simulink model "RobotArm_illinois"  (R2020a)
settings: Solver=VariableStepAuto  StartTime=0.0  StopTime=10.0  RelTol=1e-3
settings Model: Creator=nikhil  LastModifiedBy=nikhil

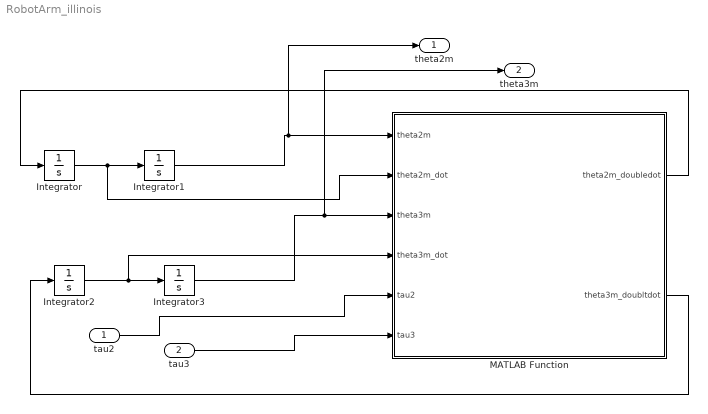
== system RobotArm_illinois ==
  tau2 : Inport
  tau3 : Inport  Port=2
  Integrator{,1..3} (4 alike) : Integrator
  MATLAB Function : MATLAB Function  TreatAsAtomicUnit=on
  theta2m : Outport
  theta3m : Outport  Port=2
  wires:
  Integrator/1 -> MATLAB Function/2(theta2m_dot), Integrator1/1
  Integrator2/1 -> MATLAB Function/4(theta3m_dot), Integrator3/1
  Integrator1/1 -> theta2m/1, MATLAB Function/1(theta2m)
  Integrator3/1 -> theta3m/1, MATLAB Function/3(theta3m)
  tau2/1 -> MATLAB Function/5(tau2)
  tau3/1 -> MATLAB Function/6(tau3)
  MATLAB Function/2(theta3m_doubltdot) -> Integrator2/1
  MATLAB Function/1(theta2m_doubledot) -> Integrator/1

== matlab function RobotArm_illinois/MATLAB Function ==
  data: theta2m input; theta2m_doubledot output; theta2m_dot input; theta3m input; theta3m_dot input; tau2 input; tau3 input; theta3m_doubltdot output
function [theta2m_doubledot, theta3m_doubltdot]  = fcn(theta2m, theta2m_dot, theta3m, theta3m_dot,tau2, tau3)
p = [0.03;0.0128;0.0076;0.0753;0.0298];
p1=p(1);
p2=p(2);
p3=p(3);
p4=p(4);
p5=p(5);
g=9.81;
Fic = [-0.04*theta2m_dot; -0.037*theta3m_dot];
tau = [tau2;tau3];
D = [p1 -p3*sin(theta3m - theta2m); -p3*sin(theta3m-theta2m) p2];
C = [0 -p3*cos(theta3m - theta2m)*theta3m_dot;
    p3*cos(theta3m-theta2m)*theta2m_dot 0];
G = [-p4*g*sin(theta2m); -p5*g*cos(theta3m)];
out = inv(D)*tau -inv(D)*C*[theta2m_dot;theta3m_dot] - inv(D)*G + inv(D)*Fic;
theta2m_doubledot = out(1);
theta3m_doubltdot = out(2);
end
